simulink model "ParameterizedMotor"  (R2015a)
settings: Solver=ode3  StartTime=0.0  StopTime=0.2  FixedStep=0.0001  RelTol=1e-3
settings Model: ExtModeTrigDuration=100  Creator=Justin  LastModifiedBy=Justin
settings OptimizationCC: OptimizeModelRefInitCode=on  LifeSpan=1
settings HardwareCC: ProdLargestAtomicInteger=Long  ProdLargestAtomicFloat=Double  ProdEndianess=LittleEndian  ProdHWDeviceType=ARM Compatible->ARM Cortex
settings RTWCC: SystemTargetFile=realtime.tlc  GenerateMakefile=off  TemplateMakefile=realtime.tmf  Description=Run on Target Hardware  RTWVerbose=off
settings ERTTargetCC: CombineOutputUpdateFcns=off  ERTSrcFileBannerTemplate=realtime_code_template.cgt  ERTHdrFileBannerTemplate=realtime_code_template.cgt  ERTDataSrcFileTemplate=realtime_code_template.cgt  ERTDataHdrFileTemplate=realtime_code_template.cgt  ERTCustomFileTemplate=realtime_file_process.tlc

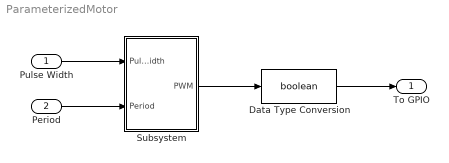
== system ParameterizedMotor ==
  Pulse Width : Inport
  Period : Inport  Port=2
  Data Type Conversion : DataTypeConversion  OutDataTypeStr=boolean
  Subsystem : Subsystem
  To GPIO : Outport
  wires:
  Data Type Conversion/1 -> To GPIO/1
  Pulse Width/1 -> Subsystem/1(Pulse Width)
  Period/1 -> Subsystem/2(Period)
  Subsystem/1(PWM) -> Data Type Conversion/1

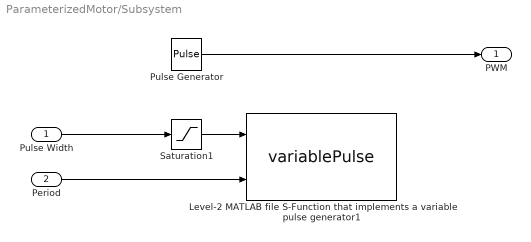
== system ParameterizedMotor/Subsystem ==
  Pulse Width : Inport
  Period : Inport  Port=2
  Level-2 MATLAB file S-Function that implements a variable pulse generator1 : M-S-Function  FunctionName=variablePulse
  Pulse Generator : DiscretePulseGenerator  PulseType=Time based  Period=0.02  PulseWidth=10
  Saturation1 : Saturate  UpperLimit=100  LowerLimit=0.1
  PWM : Outport
  wires:
  Pulse Width/1 -> Saturation1/1
  Saturation1/1 -> Level-2 MATLAB file S-Function that implements a variable pulse generator1/1
  Pulse Generator/1 -> PWM/1
  Period/1 -> Level-2 MATLAB file S-Function that implements a variable pulse generator1/2
